simulink model "NewSync_Axial_Flux_Generator_Modelled"  (R2018a)
settings: Solver=ode1  StartTime=0.0  StopTime=1  FixedStep=1e-6  MaxStep=1e-6  RelTol=1e-3
PreLoadFcn:
  | Ts=1/1000
InitFcn:
  | Pref=2000;
  | D=4;
  | P=10;
  | Rd=5;
  | Rq=5;
  | Ld=2.094;
  | Lq= 0.8187;
  | Phi= 1.6
  | Pref = 2000;
  | J=4;
  | K=0.16;
  | c1= 0.5176;
  | c2= 116;
  | c3= 0.4;
  | c4= 5;
  | c5= 21;
  | c6= 0.0068;
  | Den= 1.225;
  | A= 2
  | Ts=1/1000
undefined symbols (not defined in the file): D1, Delta
libraries: powerlib x84, powerlib_meascontrol x17, simulink x13, re_lib x1, electricdrivelib x1, pePowerMeasurement x1
(part 1 of 2)
settings Model: Creator=samue  LastModifiedBy=samue

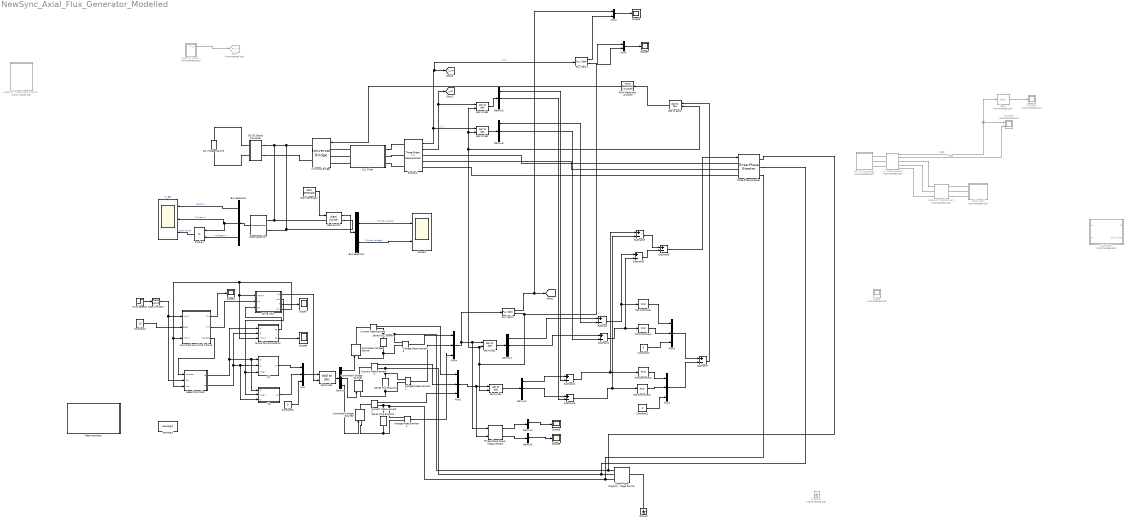
== system NewSync_Axial_Flux_Generator_Modelled ==
  AC-AC Converter : Subsystem  Commented=on
  Bus Selector1 : BusSelector  OutputSignals=SOC %,Current I,Voltage V
  Bus Selector2 : BusSelector  OutputSignals=Switch current,Switch voltage
  Busbar2 : powerlib/Measurements/Three-Phase V-I Measurement  VoltageMeasurement=phase-to-phase  SetLabelV=off  LabelV=Vabc  Vpu=off  VpuLL=off  CurrentMeasurement=yes  SetLabelI=off  LabelI=Iabc  Ipu=off  Pbase=100e6  Vbase=500e3  OutputType=Complex  PhasorSimulation=off  PSBequivalent=0
  Constant1 : Constant  Value=0
  Constant2 : Constant  Value=1.5
  Constant3 : Constant  Value=0
  Constant4 : Constant  Value=0
  Controlled Voltage Source : powerlib/Electrical Sources/Controlled Voltage Source  Initialize=on  Source_Type=AC  Amplitude=0  Phase=0  Frequency=60  Measurements=None
  Controlled Voltage Source1 : powerlib/Electrical Sources/Controlled Voltage Source  Initialize=on  Source_Type=AC  Amplitude=0  Phase=-120  Frequency=60  Measurements=None
  Controlled Voltage Source2 : powerlib/Electrical Sources/Controlled Voltage Source  Initialize=on  Source_Type=AC  Amplitude=0  Phase=120  Frequency=60  Measurements=None
  Current Measurement : powerlib/Measurements/Current Measurement  PhasorSimulation=off  OutputType=Complex  PSBequivalent=0
  Current Measurement1 : powerlib/Measurements/Current Measurement  PhasorSimulation=off  OutputType=Complex  PSBequivalent=0
  Current Measurement2 : powerlib/Measurements/Current Measurement  PhasorSimulation=off  OutputType=Complex  PSBequivalent=0
  DC Voltage Source : powerlib/Electrical Sources/DC Voltage Source  Amplitude=100  Measurements=None
  DC-DC Boost Converter : Subsystem
  Demux{,1..3,6} (5 alike) : Demux  Outputs=3
  Demux4 : Demux
  Demux5 : Demux
  Drive Train : Subsystem
  Goto : Goto  Commented=on  GotoTag=PV_m  TagVisibility=global
  Ground : powerlib/Elements/Ground  LConnTagsString=a
  Ground2 : powerlib/Elements/Ground  Commented=on  LConnTagsString=a
  Horizontal axis Wind Turbine : Subsystem
  Ideal Switch : powerlib/Power Electronics/Ideal Switch  Ron=0.001  Lon=0  IC=0  Rs=1e5  Cs=inf  Measurements=on
  Isolation Transformer1 : powerlib/Elements/Three-Phase Transformer (Two Windings)  Description=Isolation Transformer  Commented=on  Winding1Connection=Delta (D1)  Winding2Connection=Yg  CoreType=Three single-phase transformers  SetSaturation=off  Hysteresis=off  DataFile='hysteresis'  SetInitialFlux=off  Measurements=None  UNITS=pu  NominalPower=[ 1000 , 60 ]  Winding1=[ 208 , 0.002 , 0.04 ]  Winding2=[ 208 , 0.002 , 0.04 ]  Rm=200  Lm=200  L0=0.5  Saturation="[ 0,0  ;  0.005,1.2  ;  1.0,1.4 ]"  InitialFluxes=[ 0.8 , -0.8 , 0.7 ]  MoreParameters=off  BreakLoop=off  DataType=off  TransfoNumber=0
  LCL Filter : Subsystem
  Mean : powerlib_meascontrol/Measurements/Mean  Commented=on  Freq=60  Vinit=0  Ts=0
  "Measurements " : Subsystem
  Mux{,1,4..6} (5 alike) : Mux  Inputs=3
  Mux2 : Mux  Inputs=2
  Mux3 : Mux  Inputs=2
  PID Controller{,1..3} (4 alike) : simulink/Continuous/PID Controller  Controller=PI  TimeDomain=Continuous-time  SampleTime=-1  IntegratorMethod=Forward Euler  FilterMethod=Forward Euler  Form=Parallel  UseFilter=on  ControllerParametersSource=internal  P=1  I=1  D=0  N=100  InitialConditionSource=internal  InitialConditionForIntegrator=0  InitialConditionForFilter=0  ExternalReset=none  LimitOutput=off  UpperSaturationLimit=inf  LowerSaturationLimit=-inf  LinearizeAsGain=on  AntiWindupMode=none  Kb=1  TrackingMode=off  Kt=1  PParamMin=[]  PParamMax=[]  IParamMin=[]  IParamMax=[]  DParamMin=[]  DParamMax=[]  NParamMin=[]  NParamMax=[]  KbParamMin=[]  KbParamMax=[]  KtParamMin=[]  KtParamMax=[]  POutMin=[]  POutMax=[]  IOutMin=[]  IOutMax=[]  DOutMin=[]  DOutMax=[]  NOutMin=[]  NOutMax=[]  KbOutMin=[]  KbOutMax=[]  KtOutMin=[]  KtOutMax=[]  IntegratorOutMin=[]  IntegratorOutMax=[]  FilterOutMin=[]  FilterOutMax=[]  SumOutMin=[]  SumOutMax=[]  SumI1OutMin=[]  SumI1OutMax=[]  SumI2OutMin=[]  SumI2OutMax=[]  SumI3OutMin=[]  SumI3OutMax=[]  SumDOutMin=[]  SumDOutMax=[]  SaturationOutMin=[]  SaturationOutMax=[]  IntegratorContinuousStateAttributes=''  IntegratorStateMustResolveToSignalObject=off  IntegratorRTWStateStorageClass=Auto  FilterContinuousStateAttributes=''  FilterStateMustResolveToSignalObject=off  FilterRTWStateStorageClass=Auto  DifferentiatorICPrevScaledInput=0  DifferentiatorOutMin=[]  DifferentiatorOutMax=[]  FilterDiffOutCoefMin=[]  FilterDiffOutCoefMax=[]  SumDenOutMin=[]  SumDenOutMax=[]  SumNumOutMin=[]  SumNumOutMax=[]  ReciprocalOutMin=[]  ReciprocalOutMax=[]  DivideOutMin=[]  DivideOutMax=[]  TunerSelectOption=Transfer Function Based (PID Tuner App)
  PLL (3ph)1 : powerlib_meascontrol/PLL/PLL (3ph)  Fmin=45  Par_Init=[0, 60]  ParK=[180, 3200, 1]  TcD=1e-4  MaxRateChangeFreq=12  FilterCutOffFreq=25  Ts=0  AGC=on
  PLL (3ph)2 : powerlib_meascontrol/PLL/PLL (3ph)  Fmin=45  Par_Init=[0, 60]  ParK=[180, 3200, 1]  TcD=1e-4  MaxRateChangeFreq=12  FilterCutOffFreq=25  Ts=0  AGC=on
  PWM Generator (2-Level) : powerlib_meascontrol/Pulse & Signal Generators/PWM Generator (2-Level)  ModulatorType=Three-phase bridge (6 pulses)  ModulatorMode=Unsynchronized  Fc=(1000/60)*60  Pc=90  nF=27  MinMax="[ -1  1 ]"  SamplingTechnique=Natural  ModulatingSignals=off  m=0.8  Freq=60  Phase=0  Ts=(1/1000)  ShowCarrierOutport=off
      settings: SourceProductName=Simscape Power Systems
  Product : Product
  Rate Limiter2 : RateLimiter
  Scope : Scope  Commented=on
  Scope1 : Scope  NumInputPorts=2
  Scope10 : Scope  Commented=on  NumInputPorts=2
  Scope14 : Scope  Commented=on
  Scope{2..8} (7 alike) : Scope
  Series RLC Branch : powerlib/Elements/Series RLC Branch  LConnTagsString=__new0  RConnTagsString=__new0  BranchType=R  Resistance=1  Inductance=1e-3  SetiL0=off  InitialCurrent=0  Capacitance=1e-6  Setx0=off  InitialVoltage=0  Measurements=None
  Series RLC Branch1 : powerlib/Elements/Series RLC Branch  LConnTagsString=__new0  RConnTagsString=__new0  BranchType=R  Resistance=1  Inductance=1e-3  SetiL0=off  InitialCurrent=0  Capacitance=1e-6  Setx0=off  InitialVoltage=0  Measurements=None
  Series RLC Branch2 : powerlib/Elements/Series RLC Branch  LConnTagsString=__new0  RConnTagsString=__new0  BranchType=R  Resistance=1  Inductance=1e-3  SetiL0=off  InitialCurrent=0  Capacitance=1e-6  Setx0=off  InitialVoltage=0  Measurements=None
  SinePWM Three Phase Inverter : Subsystem  Commented=on
  Solar PV input1 : Subsystem  Commented=on
  Speed Controller : Subsystem
  Stair Generator : powerlib_meascontrol/Pulse & Signal Generators/Stair Generator  t=[0 3/60 8.25/60]  e=[1 0 1]  Ts=0
      settings: SourceProductName=Simscape Power Systems
  Subsystem : Subsystem  Commented=on
  Subtract{,1..7} (8 alike) : Sum  Inputs=+-
  Supercapacitor : electricdrivelib/Extra Sources/Supercapacitor  C=99.5  Rdc=8.9e-3  Voltage=48  Ns=18  Np=1  Vinit=0  Temp=25  PresetModel=off  EstParam=off  Nc=1  r=1e-9  epsilon=6.0208e-10  Ich=10  Vstern="[0.161  2.7  7.8]"  Self_dis=on  Ioc=10  Vself="[48  47.8  47.06  44.65]"  demandeplot=off  I="[10  20 100  500]"  Units=sec  Vmax=0  If=0  deltaV=0  alpha=0  sec=0
      settings: SourceProductName=Simscape Power Systems  SourceProductBaseCode=PS
  Te and Pe Computation : Subsystem
  Three-Phase Programmable Voltage Source : powerlib/Electrical Sources/Three-Phase Programmable Voltage Source  PositiveSequence="[240  0 60]"  VariationEntity=None  VariationType=Table of time-amplitude pairs  VariationTypeAlt=Step  VariationStep=0.5  VariationRate=10  VariationMagnitude=0.3  VariationFrequency=2  VariationTiming=[1 2]  VariationPhaseA=off  Amplitudes=[1 0.8 1.2 1.0]  TimeValues=[0 0.1 0.15 0.2]  HarmonicGeneration=on  HarmonicA=[3 0.2 -25 0]  HarmonicB=[2 0.15 35 2]  Timing="[0.05  3]"  BusType=swing  Pref=0  Qref=0  Qmin=-inf  Qmax=inf
  Three-Phase Breaker : powerlib/Elements/Three-Phase Breaker  InitialState=open  SwitchA=on  SwitchB=on  SwitchC=on  SwitchTimes="[1/60  5/60]"  External=on  BreakerResistance=0.01  SnubberResistance=1e6  SnubberCapacitance=inf  Measurements=None
  Three-Phase Power Measurement : pePowerMeasurement/Three-Phase Power Measurement  OverrideUsingVariant=Continuous  F=60  K=[0 1 2 3]  Seq=Positive  Ts=0
  Universal Bridge : powerlib/Power Electronics/Universal Bridge  Arms=3  SnubberResistance=1e5  SnubberCapacitance=inf  Device=IGBT / Diodes  Ron=1e-3  Lon=0  ForwardVoltages="[  0  0  ]"  ForwardVoltage=0  GTOparameters=[ 10e-6 , 20e-6 ]  IGBTparameters=[ 1e-6 , 2e-6 ]  Measurements=None  Measurements_2=None  converterType=Rectifier
  Utility Grid : Subsystem  Commented=on
  V-I measurement : powerlib/Measurements/Three-Phase V-I Measurement  Commented=on  VoltageMeasurement=phase-to-phase  SetLabelV=off  LabelV=Vinv  Vpu=off  VpuLL=off  CurrentMeasurement=yes  SetLabelI=off  LabelI=Iload  Ipu=off  Pbase=1e3  Vbase=380  OutputType=Magnitude  PhasorSimulation=off  PSBequivalent=0
  V_DC : Scope  NumInputPorts=3
  Vd : Subsystem
  Voltage Measurement1 : powerlib/Measurements/Voltage Measurement  PhasorSimulation=off  OutputType=Complex  PSBequivalent=0
  Voltage Measurement2 : powerlib/Measurements/Voltage Measurement  PhasorSimulation=off  OutputType=Complex  PSBequivalent=0
  Voltage Measurement3 : powerlib/Measurements/Voltage Measurement  PhasorSimulation=off  OutputType=Complex  PSBequivalent=0
  Vq : Subsystem
  Wind Speed2 : Step  Time=2  Before=6  After=15  SampleTime=0
  abc to dq{0..3} (4 alike) : powerlib_meascontrol/Transformations/abc to dq0  Alignment=90 degrees behind phase A axis
  dq0 to abc : powerlib_meascontrol/Transformations/dq0 to abc  Alignment=90 degrees behind phase A axis
  dq0 to abc2 : powerlib_meascontrol/Transformations/dq0 to abc  Alignment=90 degrees behind phase A axis
  powergui : powerlib/powergui  Priority=1  SimulationMode=Discrete  SampleTime=1e-6  frequency=60  Iterations=50  frequencyindice=60  Pbase=100e6  ErrMax=1e-4  UnitsV=kV  UnitsW=MW  buscounter=0  FunctionMessages=off  echomessages=off  EnableUseOfTLC=off  CurrentSourceSwitches=off  DisableSnubberDevices=off  DisableRonSwitches=off  DisableVfSwitches=off  DisplayEquations=off  SolverType=Tustin/Backward Euler (TBE)  Interpol=off  ExternalGateDelay=off  methode=off  Ts=100  x0status=blocks  SPID=on  SwTol=0  HookPort=off  RestoreLinks=warning  ResistiveCurrentMeasurement=off  Frange=[0:2:500]  Ylog=off  Xlog=on  ShowGrid=off  save=off  variable=ZData  structure=0  ZoomFFT=off  StartTime=0.0  cycles=1  DisplayStyle=1  fundamental=60  FreqAxis=off  MaxFrequency=1000  frequencyindicesteady=1  RmsSteady=1  display=off
  tag scope: Freq_Grid=global, I_inv=global, V_inv=global
  wires:
  Supercapacitor/1 -> Bus Selector1/1
  Bus Selector1/2 -> Product/1, V_DC/2  "<Current I>"
  Product/1 -> V_DC/3  "Solar Power"
  Bus Selector1/3 -> Product/2  "<Voltage V>"
  Bus Selector1/1 -> V_DC/1  "<SOC %>"
  Ideal Switch/1 -> Bus Selector2/1
  Bus Selector2/1 -> Scope1/1  "<Switch current>"
  Bus Selector2/2 -> Scope1/2  "<Switch voltage>"
  Solar PV input1/1(PV_m) -> Goto/1
  Stair Generator/1 -> Ideal Switch/1
  Demux/2 -> Controlled Voltage Source1/1
  Demux/1 -> Controlled Voltage Source/1
  dq0 to abc/1 -> Demux/1
  Horizontal axis Wind Turbine/1(Pm) -> Scope2/1
  Rate Limiter2/1 -> Speed Controller/2(Uw), Horizontal axis Wind Turbine/1(<Uw>)
  Horizontal axis Wind Turbine/2(Tm) -> Drive Train/2(Tm)
  Vd/1(vd) -> Mux/1
  Speed Controller/1(id) -> Vq/1(id), Vd/1(id), Te and Pe Computation/1(id)
  Mux/1 -> dq0 to abc/1
  Constant2/1 -> Horizontal axis Wind Turbine/2(beta)
  Drive Train/3(f) -> Scope7/1
  Demux/3 -> Controlled Voltage Source2/1
  Te and Pe Computation/2(Pe) -> Scope6/1
  Horizontal axis Wind Turbine/3(lambda) -> Speed Controller/1(lambda)
  Drive Train/4(wm) -> Speed Controller/3(Wm), Horizontal axis Wind Turbine/3(<Wm>), Drive Train/1(<Wm>), Te and Pe Computation/3(<Wm>)
  Drive Train/2(We) -> Vd/3(<We>), Vq/2(<We>)
  Vq/1(vq) -> Mux/2
  Te and Pe Computation/1(Te) -> Drive Train/3(Te)
  Drive Train/1(wt) -> dq0 to abc/2
  Wind Speed2/1 -> Rate Limiter2/1
  Speed Controller/2(iq) -> Vq/3(iq), Vd/2(iq), Te and Pe Computation/2(iq)
  Constant3/1 -> Mux/3
  Mean/1 -> Scope14/1
  V-I measurement/2 -> Scope10/2  "Iabc"
  V-I measurement/1 -> Mean/1, Scope10/1  "Vabc"
  Mux4/1 -> PLL (3ph)2/1, Three-Phase Power Measurement/1, abc to dq1/1
  Current Measurement/1 -> Mux5/1
  PLL (3ph)2/2 -> Mux3/2, dq0 to abc2/2, abc to dq3/2, abc to dq0/2, abc to dq1/2, abc to dq2/2
  Mux5/1 -> Three-Phase Power Measurement/2, abc to dq2/1
  Demux5/2 -> Scope8/1
  Demux4/2 -> Scope5/1
  Three-Phase Power Measurement/1 -> Demux4/1
  Three-Phase Power Measurement/2 -> Demux5/1
  abc to dq1/1 -> Demux1/1
  Subtract1/1 -> Subtract4/2, PID Controller1/1
  Subtract/1 -> Subtract4/1, PID Controller/1
  abc to dq2/1 -> Demux2/1
  PID Controller/1 -> Mux6/1
  PID Controller1/1 -> Mux6/2
  Constant4/1 -> Mux6/3
  Busbar2/2 -> [I_inv], abc to dq3/1  "I_inv"
  Busbar2/1 -> abc to dq0/1, PLL (3ph)1/1, [V_inv]  "V_inv"
  PLL (3ph)2/1 -> Mux2/1, [Freq_Grid]
  Current Measurement1/1 -> Mux5/2
  Voltage Measurement1/1 -> Mux4/3
  Voltage Measurement3/1 -> Mux4/1
  Voltage Measurement2/1 -> Mux4/2
  Current Measurement2/1 -> Mux5/3
  Demux1/1 -> Subtract/1
  abc to dq3/1 -> Demux3/1
  abc to dq0/1 -> Demux6/1
  Demux6/1 -> Subtract/2
  Demux1/2 -> Subtract1/1
  Demux6/2 -> Subtract1/2
  Demux2/1 -> Subtract2/1
  Demux3/1 -> Subtract2/2
  Demux2/2 -> Subtract3/1
  Demux3/2 -> Subtract3/2
  Subtract2/1 -> Subtract5/1, PID Controller2/1
  Subtract3/1 -> PID Controller3/1, Subtract5/2
  PID Controller2/1 -> Mux1/1
  PID Controller3/1 -> Mux1/2
  Constant1/1 -> Mux1/3
  Subtract5/1 -> Subtract6/1
  Subtract4/1 -> Subtract6/2
  Subtract6/1 -> Three-Phase Breaker/1
  Mux6/1 -> Subtract7/1
  Mux1/1 -> Subtract7/2
  dq0 to abc2/1 -> PWM Generator (2-Level)/1
  Subtract7/1 -> dq0 to abc2/1
  PWM Generator (2-Level)/1 -> Universal Bridge/1
  PLL (3ph)1/1 -> Mux2/2
  Mux2/1 -> Scope3/1
  PLL (3ph)1/2 -> Mux3/1
  Mux3/1 -> Scope4/1
  connections:
  Series RLC Branch1/RConn1 -- Voltage Measurement2/LConn2 -- Controlled Voltage Source1/LConn1
  Controlled Voltage Source2/LConn1 -- Voltage Measurement1/LConn2 -- Series RLC Branch2/RConn1
  Controlled Voltage Source/LConn1 -- Voltage Measurement3/LConn2 -- Series RLC Branch/RConn1
  V-I measurement/RConn2 -- Isolation Transformer1/LConn2
  Voltage Measurement1/LConn1 -- Three-Phase Breaker/RConn3 -- Three-Phase Programmable Voltage Source/RConn3 -- Current Measurement2/RConn1 -- Series RLC Branch2/LConn1
  Voltage Measurement2/LConn1 -- Three-Phase Breaker/RConn2 -- Three-Phase Programmable Voltage Source/RConn2 -- Current Measurement1/RConn1 -- Series RLC Branch1/LConn1
  V-I measurement/RConn1 -- Isolation Transformer1/LConn1
  V-I measurement/RConn3 -- Isolation Transformer1/LConn3
  Voltage Measurement3/LConn1 -- Three-Phase Breaker/RConn1 -- Three-Phase Programmable Voltage Source/RConn1 -- Current Measurement/RConn1 -- Series RLC Branch/LConn1
  LCL Filter/RConn1 -- Busbar2/LConn1
  Busbar2/LConn2 -- LCL Filter/RConn2
  Busbar2/LConn3 -- LCL Filter/RConn3
  LCL Filter/LConn1 -- Universal Bridge/LConn1
  LCL Filter/LConn2 -- Universal Bridge/LConn2
  LCL Filter/LConn3 -- Universal Bridge/LConn3
  Three-Phase Breaker/LConn1 -- Busbar2/RConn1
  Three-Phase Breaker/LConn2 -- Busbar2/RConn2
  Three-Phase Breaker/LConn3 -- Busbar2/RConn3
  Ground/LConn1 -- Three-Phase Programmable Voltage Source/LConn1
  Current Measurement2/LConn1 -- Controlled Voltage Source2/RConn1
  Current Measurement1/LConn1 -- Controlled Voltage Source1/RConn1
  Current Measurement/LConn1 -- Controlled Voltage Source/RConn1
  DC-DC Boost Converter/RConn1 -- Ideal Switch/LConn1 -- Supercapacitor/LConn1 -- Ideal Switch/RConn1 -- Supercapacitor/LConn2 -- Universal Bridge/RConn1
  DC-DC Boost Converter/RConn2 -- Universal Bridge/RConn2
  V-I measurement/LConn1 -- AC-AC Converter/RConn1
  V-I measurement/LConn2 -- AC-AC Converter/RConn2
  V-I measurement/LConn3 -- AC-AC Converter/RConn3
  Utility Grid/LConn1 -- Isolation Transformer1/RConn1
  Isolation Transformer1/RConn2 -- Utility Grid/LConn2
  Isolation Transformer1/RConn3 -- Utility Grid/LConn3
  DC Voltage Source/RConn1 -- DC-DC Boost Converter/LConn1
  DC Voltage Source/LConn1 -- DC-DC Boost Converter/LConn2

== system NewSync_Axial_Flux_Generator_Modelled/AC-AC Converter ==
  AC-DC Converter : Subsystem
  DC-AC Converter : Subsystem
  Scope : Scope
  Series RLC Branch : powerlib/Elements/Series RLC Branch  LConnTagsString=__new0  RConnTagsString=__new0  BranchType=C  Resistance=1  Inductance=1e-3  SetiL0=off  InitialCurrent=0  Capacitance=47e-6  Setx0=off  InitialVoltage=0  Measurements=None
  Voltage Measurement : powerlib/Measurements/Voltage Measurement  PhasorSimulation=off  OutputType=Complex  PSBequivalent=0
  A : PMIOPort  Side=Left
  a : PMIOPort  Port=2  Side=Right
  B : PMIOPort  Port=3  Side=Left
  b : PMIOPort  Port=4  Side=Right
  C : PMIOPort  Port=5  Side=Left
  c : PMIOPort  Port=6  Side=Right
  wires:
  Voltage Measurement/1 -> Scope/1
  connections:
  DC-AC Converter/RConn3 -- c/RConn1
  DC-AC Converter/RConn2 -- b/RConn1
  DC-AC Converter/RConn1 -- a/RConn1
  A/RConn1 -- AC-DC Converter/LConn1
  B/RConn1 -- AC-DC Converter/LConn2
  C/RConn1 -- AC-DC Converter/LConn3
  AC-DC Converter/RConn1 -- Voltage Measurement/LConn1 -- DC-AC Converter/LConn1 -- Series RLC Branch/LConn1
  AC-DC Converter/RConn2 -- Voltage Measurement/LConn2 -- DC-AC Converter/LConn2 -- Series RLC Branch/RConn1

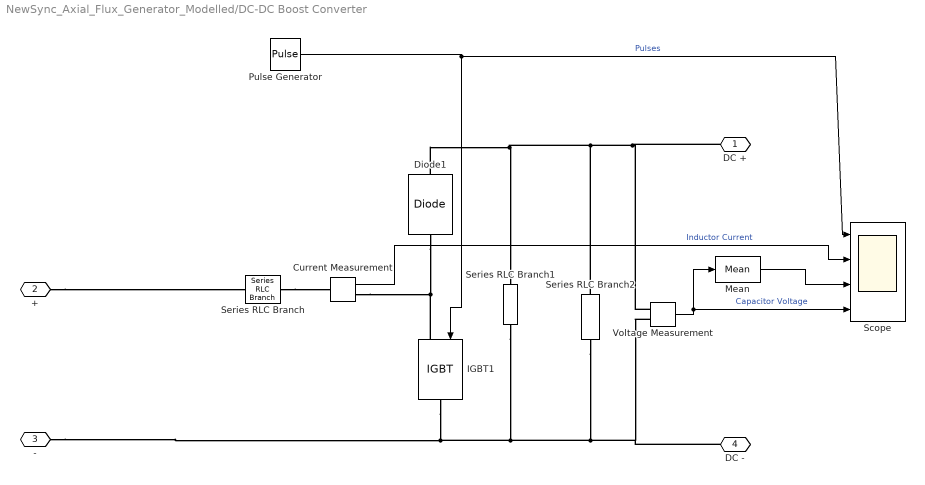
== system NewSync_Axial_Flux_Generator_Modelled/DC-DC Boost Converter ==
  Current Measurement : powerlib/Measurements/Current Measurement  PhasorSimulation=off  OutputType=Complex  PSBequivalent=0
  Diode1 : powerlib/Power Electronics/Diode  Ron=0.001  Lon=0  Vf=0.00001  IC=0  UseSnubber=0  Rs=5000000  Cs=250e-9  Measurements=off
  IGBT1 : powerlib/Power Electronics/IGBT  Ron=0.001  Lon=0  Vf=0.0001  Tf=1e-6  Tt=2e-6  IC=0  Rs=1e5  Cs=inf  Measurements=off
  Mean : powerlib_meascontrol/Measurements/Mean  Freq=60  Vinit=0  Ts=0
  Pulse Generator : DiscretePulseGenerator  PulseType=Time based  Period=1/1000  PulseWidth=50
  Scope : Scope  NumInputPorts=4
  Series RLC Branch : powerlib/Elements/Series RLC Branch  LConnTagsString=__new0  RConnTagsString=__new0  BranchType=L  Resistance=1  Inductance=200e-6  SetiL0=off  InitialCurrent=0  Capacitance=1e-6  Setx0=off  InitialVoltage=0  Measurements=None
  Series RLC Branch1 : powerlib/Elements/Series RLC Branch  LConnTagsString=__new0  RConnTagsString=__new0  BranchType=C  Resistance=1  Inductance=1e-3  SetiL0=off  InitialCurrent=0  Capacitance=100e-6  Setx0=off  InitialVoltage=0  Measurements=None
  Series RLC Branch2 : powerlib/Elements/Series RLC Branch  LConnTagsString=__new0  RConnTagsString=__new0  BranchType=R  Resistance=12  Inductance=1e-3  SetiL0=off  InitialCurrent=0  Capacitance=1e-6  Setx0=off  InitialVoltage=0  Measurements=None
  Voltage Measurement : powerlib/Measurements/Voltage Measurement  PhasorSimulation=off  OutputType=Complex  PSBequivalent=0
  DC + : PMIOPort  Side=Right
  + : PMIOPort  Port=2  Side=Left
  - : PMIOPort  Port=3  Side=Left
  DC - : PMIOPort  Port=4  Side=Right
  wires:
  Current Measurement/1 -> Scope/2  "Inductor Current"
  Voltage Measurement/1 -> Scope/4, Mean/1  "Capacitor Voltage"
  Pulse Generator/1 -> Scope/1, IGBT1/1  "Pulses"
  Mean/1 -> Scope/3
  connections:
  IGBT1/RConn1 -- -/RConn1 -- Series RLC Branch1/RConn1 -- Voltage Measurement/LConn2 -- DC -/RConn1 -- Series RLC Branch2/RConn1
  Voltage Measurement/LConn1 -- DC +/RConn1 -- Series RLC Branch2/LConn1 -- Diode1/RConn1 -- Series RLC Branch1/LConn1
  Diode1/LConn1 -- IGBT1/LConn1 -- Current Measurement/RConn1
  Series RLC Branch/RConn1 -- Current Measurement/LConn1
  +/RConn1 -- Series RLC Branch/LConn1

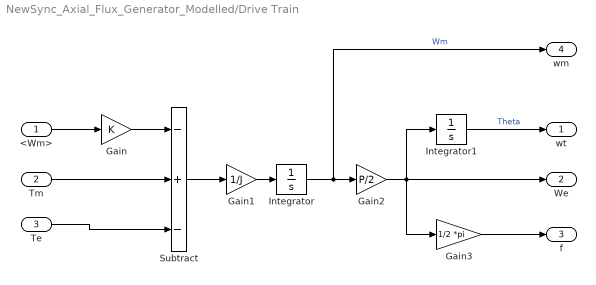
== system NewSync_Axial_Flux_Generator_Modelled/Drive Train ==
  <Wm> : Inport
  Tm : Inport  Port=2
  Te : Inport  Port=3
  Gain : Gain  Gain=K
  Gain1 : Gain  Gain=1/J
  Gain2 : Gain  Gain=P/2
  Gain3 : Gain  Gain=1/2 *pi
  Integrator : Integrator
  Integrator1 : Integrator
  Subtract : Sum  Inputs=-+-
  wt : Outport
  We : Outport  Port=2
  f : Outport  Port=3
  wm : Outport  Port=4
  wires:
  Tm/1 -> Subtract/2
  Integrator/1 -> wm/1, Gain2/1  "Wm"
  Gain/1 -> Subtract/1
  Gain2/1 -> We/1, Integrator1/1, Gain3/1
  Te/1 -> Subtract/3
  <Wm>/1 -> Gain/1
  Gain1/1 -> Integrator/1
  Subtract/1 -> Gain1/1
  Integrator1/1 -> wt/1  "Theta"
  Gain3/1 -> f/1

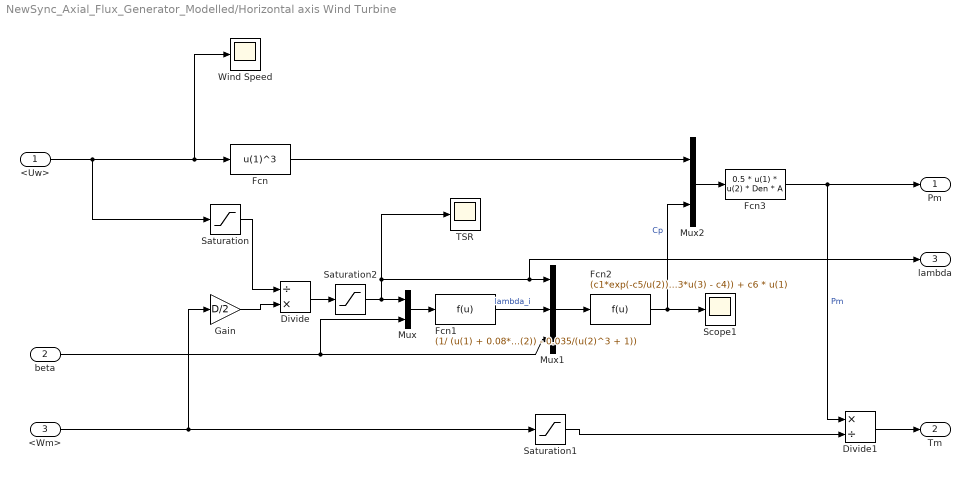
== system NewSync_Axial_Flux_Generator_Modelled/Horizontal axis Wind Turbine ==
  <Uw> : Inport
  beta : Inport  Port=2
  <Wm> : Inport  Port=3
  Divide : Product  Inputs=/*
  Divide1 : Product  Inputs=*/
  Fcn : Fcn  Expr=u(1)^3
  Fcn1 : Fcn  Expr=(1/ (u(1) + 0.08*u(2)) - 0.035/(u(2)^3 + 1))
  Fcn2 : Fcn  Expr=(c1*exp(-c5/u(2))*(c2/u(2) - c3*u(3) - c4)) + c6 * u(1)
  Fcn3 : Fcn  Expr=0.5 * u(1) * u(2) * Den * A
  Gain : Gain  Gain=D/2
  Mux : Mux  Inputs=2
  Mux1 : Mux  Inputs=3
  Mux2 : Mux  Inputs=2
  Saturation : Saturate
  Saturation1 : Saturate  UpperLimit=1e6  LowerLimit=1e-6
  Saturation2 : Saturate  UpperLimit=inf  LowerLimit=1e-6
  Scope1 : Scope
  TSR : Scope
  Wind Speed : Scope
  Pm : Outport
  Tm : Outport  Port=2
  lambda : Outport  Port=3
  wires:
  beta/1 -> Mux/2, Mux1/3
  Fcn2/1 -> Scope1/1, Mux2/2  "Cp"
  Divide/1 -> Saturation2/1
  Saturation2/1 -> Mux/1, lambda/1, Mux1/1, TSR/1
  Gain/1 -> Divide/2
  Fcn3/1 -> Pm/1, Divide1/1  "Pm"
  <Uw>/1 -> Saturation/1, Wind Speed/1, Fcn/1
  Mux/1 -> Fcn1/1
  Saturation1/1 -> Divide1/2
  Fcn1/1 -> Mux1/2  "lambda_i"
  <Wm>/1 -> Saturation1/1, Gain/1
  Mux1/1 -> Fcn2/1
  Mux2/1 -> Fcn3/1
  Fcn/1 -> Mux2/1
  Divide1/1 -> Tm/1
  Saturation/1 -> Divide/1

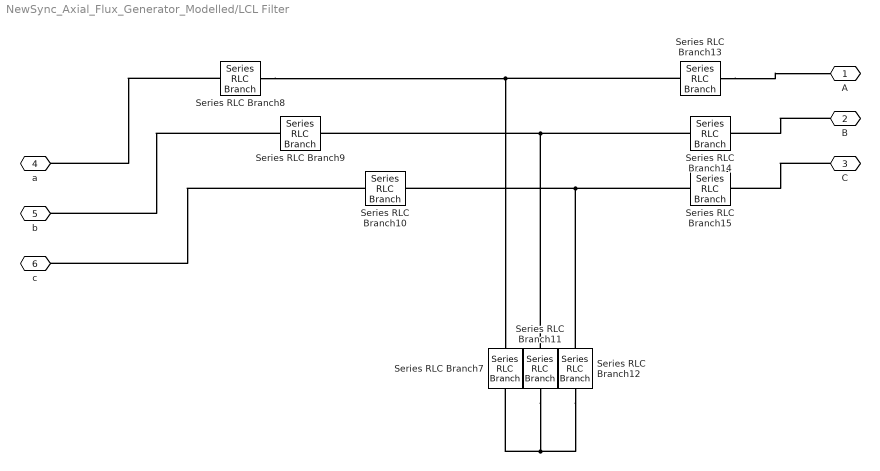
== system NewSync_Axial_Flux_Generator_Modelled/LCL Filter ==
  Series RLC Branch{8..10,13..15} (6 alike) : powerlib/Elements/Series RLC Branch  LConnTagsString=__new0  RConnTagsString=__new0  BranchType=L  Resistance=1  Inductance=20e-3  SetiL0=off  InitialCurrent=0  Capacitance=1e-6  Setx0=off  InitialVoltage=0  Measurements=None
  Series RLC Branch11 : powerlib/Elements/Series RLC Branch  LConnTagsString=__new0  RConnTagsString=__new0  BranchType=C  Resistance=1  Inductance=1e-3  SetiL0=off  InitialCurrent=0  Capacitance=100e-6  Setx0=off  InitialVoltage=0  Measurements=None
  Series RLC Branch12 : powerlib/Elements/Series RLC Branch  LConnTagsString=__new0  RConnTagsString=__new0  BranchType=C  Resistance=1  Inductance=1e-3  SetiL0=off  InitialCurrent=0  Capacitance=100e-6  Setx0=off  InitialVoltage=0  Measurements=None
  Series RLC Branch7 : powerlib/Elements/Series RLC Branch  LConnTagsString=__new0  RConnTagsString=__new0  BranchType=C  Resistance=1  Inductance=1e-3  SetiL0=off  InitialCurrent=0  Capacitance=100e-6  Setx0=off  InitialVoltage=0  Measurements=None
  A : PMIOPort  Side=Right
  B : PMIOPort  Port=2  Side=Right
  C : PMIOPort  Port=3  Side=Right
  a : PMIOPort  Port=4  Side=Left
  b : PMIOPort  Port=5  Side=Left
  c : PMIOPort  Port=6  Side=Left
  connections:
  Series RLC Branch12/LConn1 -- Series RLC Branch10/RConn1 -- Series RLC Branch15/LConn1
  Series RLC Branch12/RConn1 -- Series RLC Branch7/RConn1 -- Series RLC Branch11/RConn1
  Series RLC Branch13/RConn1 -- A/RConn1
  Series RLC Branch9/LConn1 -- b/RConn1
  Series RLC Branch8/RConn1 -- Series RLC Branch13/LConn1 -- Series RLC Branch7/LConn1
  Series RLC Branch11/LConn1 -- Series RLC Branch14/LConn1 -- Series RLC Branch9/RConn1
  Series RLC Branch10/LConn1 -- c/RConn1
  Series RLC Branch8/LConn1 -- a/RConn1
  C/RConn1 -- Series RLC Branch15/RConn1
  B/RConn1 -- Series RLC Branch14/RConn1

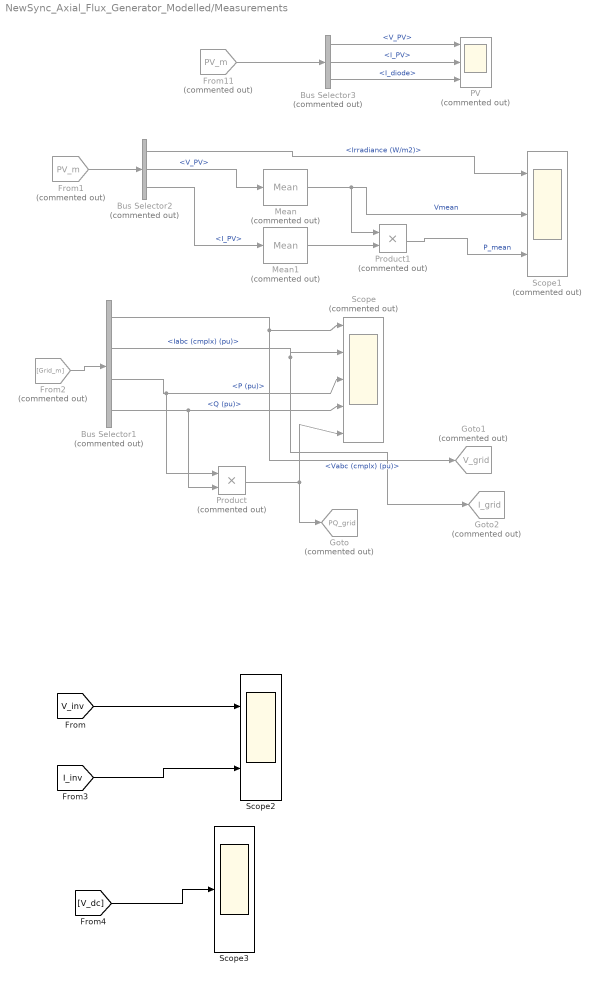
== system NewSync_Axial_Flux_Generator_Modelled/Measurements  ==
  Bus Selector1 : BusSelector  Commented=on  OutputSignals=Vabc (cmplx) (pu),Iabc (cmplx) (pu),P (pu),Q (pu)
  Bus Selector2 : BusSelector  Commented=on  OutputSignals=Irradiance (W/m2),V_PV,I_PV
  Bus Selector3 : BusSelector  Commented=on  OutputSignals=V_PV,I_PV,I_diode
  From1 : From  Commented=on  GotoTag=PV_m
  From11 : From  Commented=on  GotoTag=PV_m
  From2 : From  Commented=on  GotoTag=Grid_m
  Goto : Goto  Commented=on  GotoTag=PQ_grid  TagVisibility=global
  Goto1 : Goto  Commented=on  GotoTag=V_grid  TagVisibility=global
  Goto2 : Goto  Commented=on  GotoTag=I_grid  TagVisibility=global
  Mean : powerlib_meascontrol/Measurements/Mean  Commented=on  Freq=60  Vinit=406  Ts=0
  Mean1 : powerlib_meascontrol/Measurements/Mean  Commented=on  Freq=60  Vinit=8.05  Ts=0
  PV : Scope  Commented=on  NumInputPorts=3
  Product : Product  Commented=on
  Product1 : Product  Commented=on
  Scope : Scope  Commented=on  NumInputPorts=5
  Scope1 : Scope  Commented=on  NumInputPorts=3
  Scope2 : Scope  NumInputPorts=2
  Scope3 : Scope
  wires:
  From2/1 -> Bus Selector1/1
  Bus Selector1/1 -> Goto1/1, Scope/1  "<Vabc (cmplx) (pu)>"
  Bus Selector1/2 -> Goto2/1, Scope/2  "<Iabc (cmplx) (pu)>"
  Bus Selector1/3 -> Product/1, Scope/3  "<P (pu)>"
  Bus Selector1/4 -> Product/2, Scope/4  "<Q (pu)>"
  Product/1 -> Scope/5, Goto/1
  Bus Selector2/1 -> Scope1/1  "<Irradiance (W/m2)>"
  Bus Selector2/3 -> Mean1/1  "<I_PV>"
  Product1/1 -> Scope1/3  "P_mean"
  Mean/1 -> Scope1/2, Product1/1  "Vmean"
  Mean1/1 -> Product1/2
  From1/1 -> Bus Selector2/1
  Bus Selector2/2 -> Mean/1  "<V_PV>"
  Bus Selector3/3 -> PV/3  "<I_diode>"
  Bus Selector3/2 -> PV/2  "<I_PV>"
  Bus Selector3/1 -> PV/1  "<V_PV>"
  From11/1 -> Bus Selector3/1
  [V_inv] -> Scope2/1
  [I_inv] -> Scope2/2
  [V_dc] -> Scope3/1

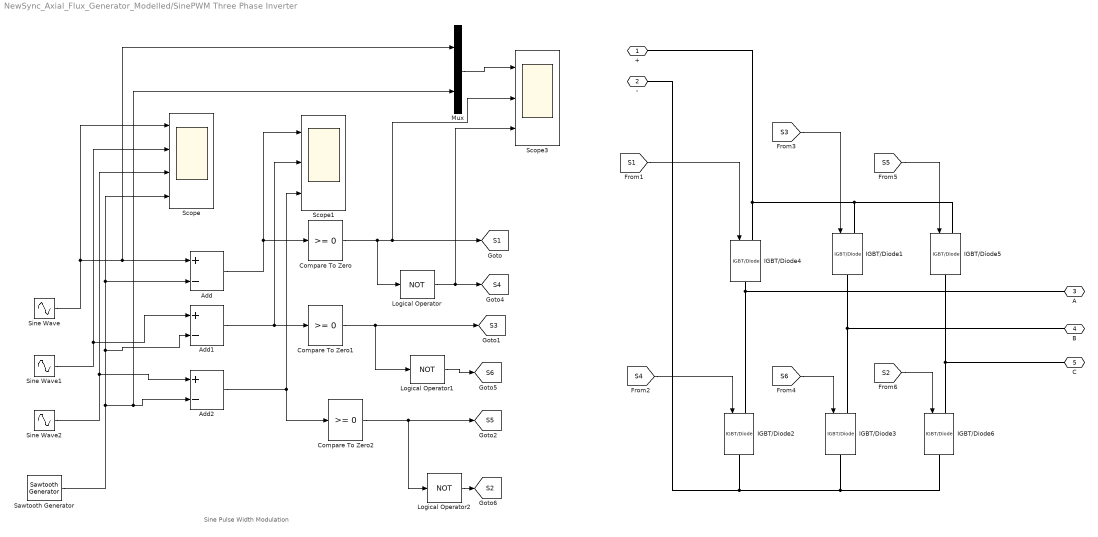
== system NewSync_Axial_Flux_Generator_Modelled/SinePWM Three Phase Inverter ==
  note: Sine Pulse Width Modulation
  Add : Sum  Inputs=+-
  Add1 : Sum  Inputs=+-
  Add2 : Sum  Inputs=+-
  Compare To Zero : simulink/Logic and Bit Operations/Compare To Zero  relop=>=  OutDataTypeStr=boolean
  Compare To Zero1 : simulink/Logic and Bit Operations/Compare To Zero  relop=>=  OutDataTypeStr=boolean
  Compare To Zero2 : simulink/Logic and Bit Operations/Compare To Zero  relop=>=  OutDataTypeStr=boolean
  IGBT/Diode{1..6} (6 alike) : powerlib/Power Electronics/IGBT//Diode  Ron=1e-3  Rs=1e5  Cs=inf  Measurements=off
  Logical Operator : Logic  Operator=NOT  AllPortsSameDT=off  OutDataTypeStr=boolean
  Logical Operator1 : Logic  Operator=NOT  AllPortsSameDT=off  OutDataTypeStr=boolean
  Logical Operator2 : Logic  Operator=NOT  AllPortsSameDT=off  OutDataTypeStr=boolean
  Mux : Mux  Inputs=2
  Sawtooth Generator : powerlib_meascontrol/Pulse & Signal Generators/Sawtooth Generator  Freq=10  Phase=180  Ts=0
      settings: SourceProductName=Simscape Power Systems
  Scope : Scope  NumInputPorts=4
  Scope1 : Scope  NumInputPorts=3
  Scope3 : Scope  NumInputPorts=3
  Sine Wave : Sin  Frequency=2*pi*60  SampleTime=0
  Sine Wave1 : Sin  Frequency=2*pi*60  Phase=(2*pi)/3  SampleTime=0
  Sine Wave2 : Sin  Frequency=2*pi*60  Phase=(-2*pi)/3  SampleTime=0
  + : PMIOPort  Side=Left
  - : PMIOPort  Port=2  Side=Left
  A : PMIOPort  Port=3  Side=Right
  B : PMIOPort  Port=4  Side=Right
  C : PMIOPort  Port=5  Side=Right
  tag scope: S1=global, S2=global, S3=global, S4=global, S5=global, S6=global
  wires:
  Sawtooth Generator/1 -> Mux/2, Add2/2, Add1/2, Add/2, Scope/4
  Add/1 -> Scope1/1, Compare To Zero/1
  Add1/1 -> Compare To Zero1/1, Scope1/2
  Compare To Zero/1 -> [S1], Scope3/2, Logical Operator/1
  [S6] -> IGBT/Diode3/1
  Compare To Zero1/1 -> Logical Operator1/1, [S3]
  Sine Wave/1 -> Mux/1, Add/1, Scope/1
  Sine Wave2/1 -> Add2/1, Scope/3
  Mux/1 -> Scope3/1
  Compare To Zero2/1 -> Logical Operator2/1, [S5]
  [S2] -> IGBT/Diode6/1
  [S1] -> IGBT/Diode4/1
  [S3] -> IGBT/Diode1/1
  [S4] -> IGBT/Diode2/1
  [S5] -> IGBT/Diode5/1
  Add2/1 -> Compare To Zero2/1, Scope1/3
  Sine Wave1/1 -> Add1/1, Scope/2
  Logical Operator2/1 -> [S2]
  Logical Operator1/1 -> [S6]
  Logical Operator/1 -> Scope3/3, [S4]
  connections:
  IGBT/Diode6/LConn1 -- C/RConn1 -- IGBT/Diode5/RConn1
  IGBT/Diode4/RConn1 -- IGBT/Diode2/LConn1 -- A/RConn1
  IGBT/Diode4/LConn1 -- +/RConn1 -- IGBT/Diode5/LConn1 -- IGBT/Diode1/LConn1
  IGBT/Diode6/RConn1 -- -/RConn1 -- IGBT/Diode2/RConn1 -- IGBT/Diode3/RConn1
  IGBT/Diode3/LConn1 -- B/RConn1 -- IGBT/Diode1/RConn1

== system NewSync_Axial_Flux_Generator_Modelled/Solar PV input1 ==
  Display1 : Display
  Display2 : Display
  Environment Temperature : UniformRandomNumber  Minimum=5  Maximum=55  SampleTime=0
  Irradiance : UniformRandomNumber  Minimum=700  Maximum=1200  SampleTime=0
  PV Array : re_lib/Solar/PV Array  Npar=1  Nser=14  PlotType=array @ 1000 W/m2 & specified temperatures  S_vec="[ 1000  500  100 ]"  Temp_C_vec=[ 45 25 100 ]  ModuleName=1Soltech 1STH-245-WH  PlotWhenSelected=off  Pm=244.62  Ncell=60  Voc=37.2  Isc=8.62  Vm=30.2  Im=8.1  beta_Voc_pc=-0.36901  alpha_Isc_pc=0.086995  beta_Voc=-0.13727  alpha_Isc=0.007499  IL=8.6566  I0=4.1387e-10  nI=1.0162  Rsh=269.0242  Rs=0.29571  BAL=on  Tc=1e-6  Tfilter=5e-5
      settings: AttributesFormatString=|
      | %<ModuleName>
      | %<Nser>-module string
      | %<Npar> parallel strings
  Rate Limiter1 : RateLimiter  RisingSlewLimit=8000  FallingSlewLimit=-8000  InitialCondition=1000
  Saturation : Saturate  UpperLimit=55  LowerLimit=5
  + : PMIOPort  Side=Right
  - : PMIOPort  Port=2  Side=Right
  PV_m : Outport
  wires:
  Rate Limiter1/1 -> Display2/1, PV Array/1
  Environment Temperature/1 -> Saturation/1
  Irradiance/1 -> Rate Limiter1/1
  PV Array/1 -> PV_m/1
  Saturation/1 -> Display1/1, PV Array/2
  connections:
  PV Array/RConn2 -- -/RConn1
  PV Array/RConn1 -- +/RConn1

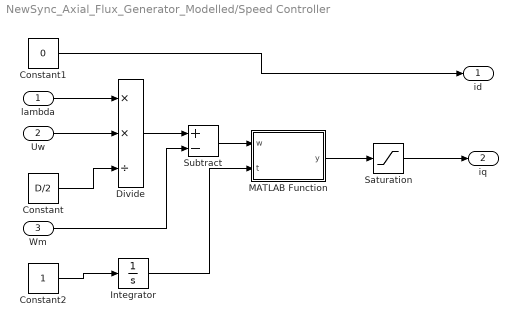
== system NewSync_Axial_Flux_Generator_Modelled/Speed Controller ==
  lambda : Inport
  Uw : Inport  Port=2
  Wm : Inport  Port=3
  Constant : Constant  Value=D/2
  Constant1 : Constant  Value=0
  Constant2 : Constant
  Divide : Product  Inputs=**/
  Integrator : Integrator
  MATLAB Function : MATLAB Function  TreatAsAtomicUnit=on
  Saturation : Saturate
  Subtract : Sum  Inputs=+-
  id : Outport
  iq : Outport  Port=2
  wires:
  MATLAB Function/1(y) -> Saturation/1
  Divide/1 -> Subtract/1
  Integrator/1 -> MATLAB Function/2(t)
  Saturation/1 -> iq/1
  Constant2/1 -> Integrator/1
  Constant/1 -> Divide/3
  Wm/1 -> Subtract/2
  Uw/1 -> Divide/2
  Constant1/1 -> id/1
  Subtract/1 -> MATLAB Function/1(w)
  lambda/1 -> Divide/1

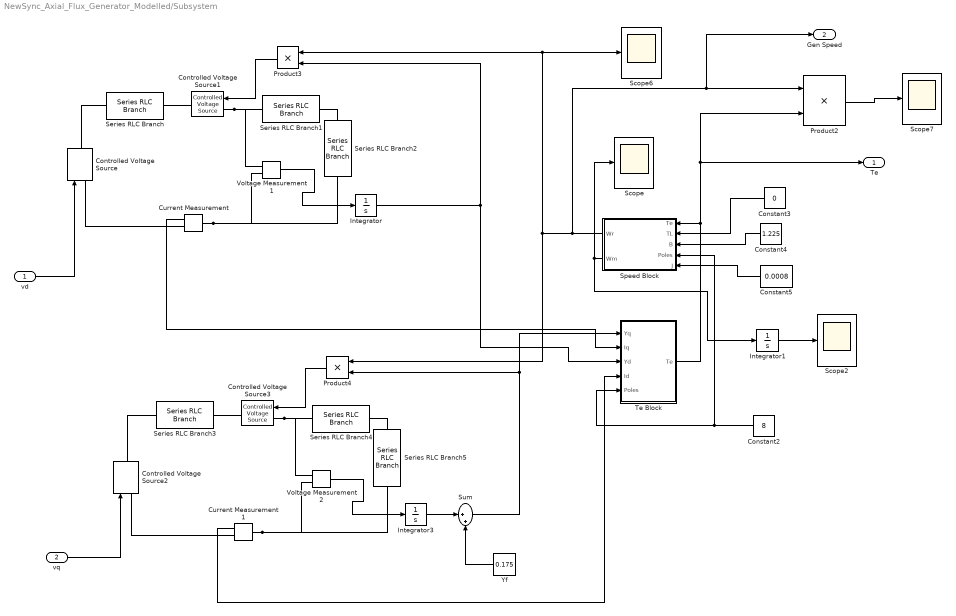
== system NewSync_Axial_Flux_Generator_Modelled/Subsystem ==
  vd : Inport
  vq : Inport  Port=2
  Constant2 : Constant  Value=8
  Constant3 : Constant  Value=0
  Constant4 : Constant  Value=1.225
  Constant5 : Constant  Value=0.0008
  Controlled Voltage Source{,1..3} (4 alike) : powerlib/Electrical Sources/Controlled Voltage Source  Initialize=on  Source_Type=AC  Amplitude=0  Phase=0  Frequency=0  Measurements=None
  Current Measurement : powerlib/Measurements/Current Measurement  PhasorSimulation=off  OutputType=Complex  PSBequivalent=0
  Current Measurement1 : powerlib/Measurements/Current Measurement  PhasorSimulation=off  OutputType=Complex  PSBequivalent=0
  Integrator : Integrator
  Integrator1 : Integrator
  Integrator3 : Integrator
  Product2 : Product
  Product3 : Product
  Product4 : Product
  Scope{,2,6..7} (4 alike) : Scope
  Series RLC Branch : powerlib/Elements/Series RLC Branch  LConnTagsString=__new0  RConnTagsString=__new0  BranchType=R  Resistance=2.875  Inductance=1e-3  SetiL0=off  InitialCurrent=0  Capacitance=1e-6  Setx0=off  InitialVoltage=0  Measurements=None
  Series RLC Branch1 : powerlib/Elements/Series RLC Branch  LConnTagsString=__new0  RConnTagsString=__new0  BranchType=L  Resistance=1  Inductance=9e-3  SetiL0=off  InitialCurrent=0  Capacitance=1e-6  Setx0=off  InitialVoltage=0  Measurements=None
  Series RLC Branch2 : powerlib/Elements/Series RLC Branch  LConnTagsString=__new0  RConnTagsString=__new0  BranchType=L  Resistance=1  Inductance=9e-3  SetiL0=off  InitialCurrent=0  Capacitance=1e-6  Setx0=off  InitialVoltage=0  Measurements=None
  Series RLC Branch3 : powerlib/Elements/Series RLC Branch  LConnTagsString=__new0  RConnTagsString=__new0  BranchType=R  Resistance=2.875  Inductance=1e-3  SetiL0=off  InitialCurrent=0  Capacitance=1e-6  Setx0=off  InitialVoltage=0  Measurements=None
  Series RLC Branch4 : powerlib/Elements/Series RLC Branch  LConnTagsString=__new0  RConnTagsString=__new0  BranchType=L  Resistance=1  Inductance=7e-3  SetiL0=off  InitialCurrent=0  Capacitance=1e-6  Setx0=off  InitialVoltage=0  Measurements=None
  Series RLC Branch5 : powerlib/Elements/Series RLC Branch  LConnTagsString=__new0  RConnTagsString=__new0  BranchType=L  Resistance=1  Inductance=7e-3  SetiL0=off  InitialCurrent=0  Capacitance=1e-6  Setx0=off  InitialVoltage=0  Measurements=None
  Speed Block : Subsystem
  Sum : Sum  Inputs=|++
  Te Block : Subsystem
  Voltage Measurement1 : powerlib/Measurements/Voltage Measurement  PhasorSimulation=off  OutputType=Complex  PSBequivalent=0
  Voltage Measurement2 : powerlib/Measurements/Voltage Measurement  PhasorSimulation=off  OutputType=Complex  PSBequivalent=0
  Yf : Constant  Value=0.175
  Te : Outport
  Gen Speed : Outport  Port=2
  wires:
  Constant2/1 -> Te Block/5(Poles), Speed Block/4(Poles)
  Speed Block/2(Wm) -> Integrator1/1, Scope/1
  Product3/1 -> Controlled Voltage Source1/1
  Te Block/1(Te) -> Te/1, Product2/2, Speed Block/1(Te)
  Sum/1 -> Product4/2, Te Block/1(Yq)
  Integrator/1 -> Product3/2, Te Block/3(Yd)
  Speed Block/1(Wr) -> Gen Speed/1, Product2/1, Scope6/1, Product3/1, Product4/1
  Integrator1/1 -> Scope2/1
  Voltage Measurement2/1 -> Integrator3/1
  Voltage Measurement1/1 -> Integrator/1
  Constant4/1 -> Speed Block/3(B)
  vq/1 -> Controlled Voltage Source2/1
  Current Measurement1/1 -> Te Block/4(Id)
  Yf/1 -> Sum/2
  Product4/1 -> Controlled Voltage Source3/1
  Integrator3/1 -> Sum/1
  Constant5/1 -> Speed Block/5(J)
  Product2/1 -> Scope7/1
  Current Measurement/1 -> Te Block/2(Iq)
  Constant3/1 -> Speed Block/2(TL)
  vd/1 -> Controlled Voltage Source/1
  connections:
  Controlled Voltage Source1/LConn1 -- Voltage Measurement1/LConn1 -- Series RLC Branch1/LConn1
  Series RLC Branch2/LConn1 -- Series RLC Branch1/RConn1
  Controlled Voltage Source3/RConn1 -- Series RLC Branch3/RConn1
  Series RLC Branch/LConn1 -- Controlled Voltage Source/RConn1
  Controlled Voltage Source3/LConn1 -- Voltage Measurement2/LConn1 -- Series RLC Branch4/LConn1
  Controlled Voltage Source1/RConn1 -- Series RLC Branch/RConn1
  Current Measurement1/RConn1 -- Controlled Voltage Source2/LConn1
  Current Measurement1/LConn1 -- Series RLC Branch5/RConn1 -- Voltage Measurement2/LConn2
  Current Measurement/LConn1 -- Series RLC Branch2/RConn1 -- Voltage Measurement1/LConn2
  Series RLC Branch3/LConn1 -- Controlled Voltage Source2/RConn1
  Current Measurement/RConn1 -- Controlled Voltage Source/LConn1
  Series RLC Branch5/LConn1 -- Series RLC Branch4/RConn1

== system NewSync_Axial_Flux_Generator_Modelled/Te and Pe Computation ==
  id : Inport
  iq : Inport  Port=2
  <Wm> : Inport  Port=3
  Gain : Gain  Gain=Ld-Lq
  Gain1 : Gain  Gain=Phi
  Gain2 : Gain  Gain=0.75*P
  Product : Product
  Product1 : Product
  Sum : Sum  Inputs=|-+
  Te : Outport
  Pe : Outport  Port=2
  wires:
  <Wm>/1 -> Product1/2
  Product/1 -> Gain/1
  Sum/1 -> Gain2/1
  Gain/1 -> Sum/1
  Gain2/1 -> Te/1, Product1/1  "Te"
  Gain1/1 -> Sum/2
  Product1/1 -> Pe/1
  iq/1 -> Gain1/1, Product/2
  id/1 -> Product/1
